simulink model "e2_1"  (R2022a)
settings: Solver=VariableStepAuto  StartTime=0.0  StopTime=50  MaxStep=0.1  RelTol=1e-3  AbsTol=1e-6
settings Model: Creator=18075  LastModifiedBy=18075

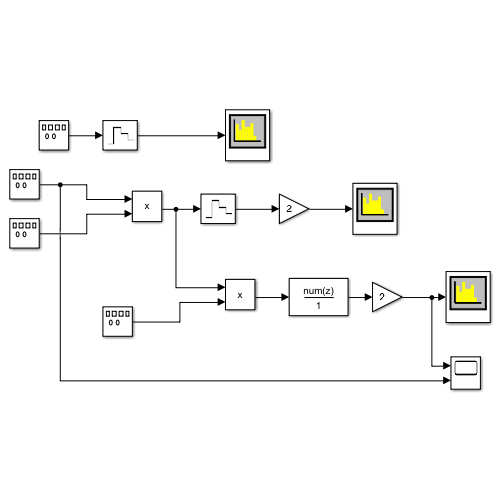
[thumbnail: Simulink's stored preview of the top-level diagram]
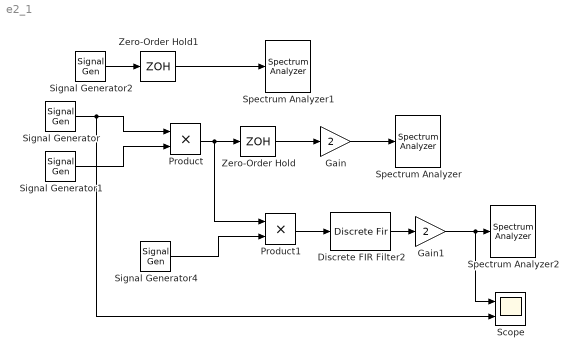
== system e2_1 ==
  Discrete FIR Filter2 : DiscreteFir  Coefficients=fir1(16,0.2,hanning(17))
  Gain : Gain  Gain=2
  Gain1 : Gain  Gain=2
  Product : Product
  Product1 : Product
  Scope : Scope  NumInputPorts=2
  Signal Generator : SignalGenerator  WaveForm=sawtooth
  Signal Generator1 : SignalGenerator  Frequency=10000
  Signal Generator2 : SignalGenerator  WaveForm=sawtooth
  Signal Generator4 : SignalGenerator  Frequency=10000
  Spectrum Analyzer : SpectrumAnalyzer
  Spectrum Analyzer1 : SpectrumAnalyzer
  Spectrum Analyzer2 : SpectrumAnalyzer
  Zero-Order Hold : ZeroOrderHold  SampleTime=-1
  Zero-Order Hold1 : ZeroOrderHold  SampleTime=-1
  wires:
  Signal Generator/1 -> Scope/2, Product/1
  Signal Generator1/1 -> Product/2
  Product/1 -> Zero-Order Hold/1, Product1/1
  Zero-Order Hold/1 -> Gain/1
  Gain/1 -> Spectrum Analyzer/1
  Zero-Order Hold1/1 -> Spectrum Analyzer1/1
  Signal Generator2/1 -> Zero-Order Hold1/1
  Gain1/1 -> Scope/1, Spectrum Analyzer2/1
  Signal Generator4/1 -> Product1/2
  Discrete FIR Filter2/1 -> Gain1/1
  Product1/1 -> Discrete FIR Filter2/1
